simulink model "accel_test"  (R2022a)
settings: Solver=VariableStepAuto  StartTime=0.0  StopTime=10.0  RelTol=1e-3
values from neighbouring files (symbols this model uses):
  nx = 12 + 2*n    [nmpc_matlab.m]    (also in nmpc_test.m)
  ny = 8    [nmpc_matlab.m]    (also in nmpc_test.m)
  q_dot_0 = zeros(N, 1)    [ee_dyn_check.m]
  tau = [taub; taum]    [ee_dyn_check.m]
undefined symbols (not defined in the file or in its folder): fx, fy, fz, nz, q_0
settings Model: Creator=charl  LastModifiedBy=charl

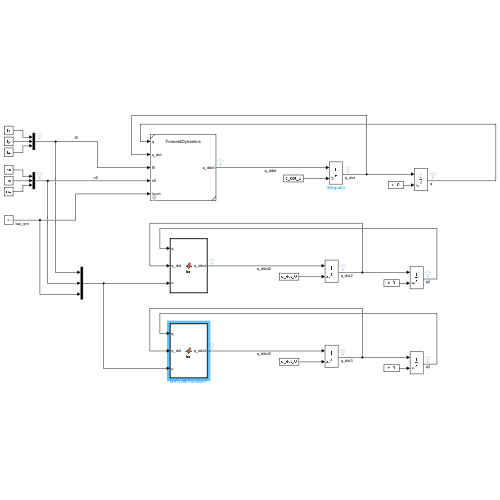
[thumbnail: Simulink's stored preview of the top-level diagram]
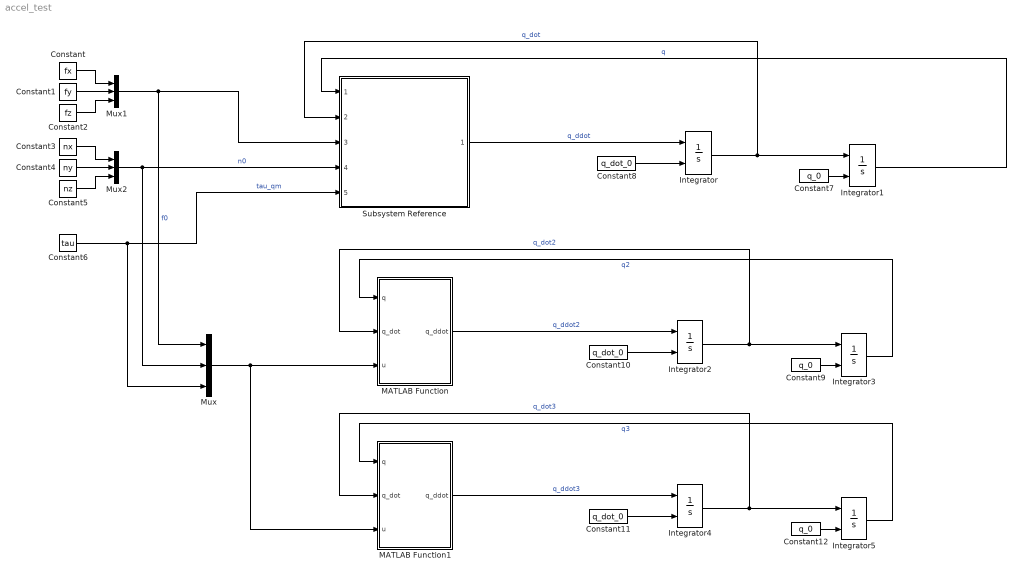
== system accel_test ==
  Constant : Constant  Value=fx
  Constant1 : Constant  Value=fy
  Constant10 : Constant  Value=q_dot_0
  Constant11 : Constant  Value=q_dot_0
  Constant12 : Constant  Value=q_0
  Constant2 : Constant  Value=fz
  Constant3 : Constant  Value=nx
  Constant4 : Constant  Value=ny
  Constant5 : Constant  Value=nz
  Constant6 : Constant  Value=tau
  Constant7 : Constant  Value=q_0
  Constant8 : Constant  Value=q_dot_0
  Constant9 : Constant  Value=q_0
  Integrator{,1..5} (6 alike) : Integrator  InitialConditionSource=external
  MATLAB Function : MATLAB Function  TreatAsAtomicUnit=on
  MATLAB Function1 : MATLAB Function  TreatAsAtomicUnit=on
  Mux : Mux  Inputs=3
  Mux1 : Mux  Inputs=3
  Mux2 : Mux  Inputs=3
  Subsystem Reference : Subsystem  ReferencedSubsystem=ForwardDynamics  spaceRobot=sr  SimulateUsing=Interpreted execution
  wires:
  Integrator/1 -> Subsystem Reference/2, Integrator1/1  "q_dot"
  Integrator1/1 -> Subsystem Reference/1  "q"
  Constant7/1 -> Integrator1/2
  Constant8/1 -> Integrator/2
  Subsystem Reference/1 -> Integrator/1  "q_ddot"
  Mux1/1 -> Mux/1, Subsystem Reference/3  "f0"
  Constant4/1 -> Mux2/2
  Mux2/1 -> Mux/2, Subsystem Reference/4  "n0"
  Constant/1 -> Mux1/1
  Constant6/1 -> Mux/3, Subsystem Reference/5  "tau_qm"
  Constant2/1 -> Mux1/3
  Constant1/1 -> Mux1/2
  Constant3/1 -> Mux2/1
  Constant5/1 -> Mux2/3
  MATLAB Function/1(q_ddot) -> Integrator2/1  "q_ddot2"
  Constant9/1 -> Integrator3/2
  Integrator2/1 -> MATLAB Function/2(q_dot), Integrator3/1  "q_dot2"
  Integrator3/1 -> MATLAB Function/1(q)  "q2"
  Constant10/1 -> Integrator2/2
  Constant12/1 -> Integrator5/2
  MATLAB Function1/1(q_ddot) -> Integrator4/1  "q_ddot3"
  Integrator5/1 -> MATLAB Function1/1(q)  "q3"
  Mux/1 -> MATLAB Function1/3(u), MATLAB Function/3(u)
  Constant11/1 -> Integrator4/2
  Integrator4/1 -> MATLAB Function1/2(q_dot), Integrator5/1  "q_dot3"

== matlab function accel_test/MATLAB Function1 ==
  data: q input; q_ddot output; q_dot input; u input
function q_ddot = fcn(q, q_dot, u)

%% Load params
sr_info = SR2_info();

%%
% 1 - Kinematics
[Rb, Ra, Rm] = RFunc_SR2(q);
Rm = reshape(Rm, 3, 3, []); % Split Rm to nk 3x3 arrays

% 2 - Kinetics
[t, ~, Omega, A, A_dot] = Kin(sr_info, q, q_dot, zeros(8, 1), {Rb, Ra, Rm});

% 3 - ID  
wb = t{1}(4:6);
C = CorMat(sr_info, wb, Omega, A, A_dot, {Rb, Ra, Rm});
h = C*q_dot;

% 4 - Mass Mat
D = MassM(sr_info, q, A);

% 5 - FD
q_ddot = D^ - 1 * (u - h);

== matlab function accel_test/MATLAB Function ==
  data: q input; q_ddot output; q_dot input; u input
function q_ddot = fcn(q, q_dot, u)

%% Load params
sr_info = SR2_info();

%%
% 1 - Kinematics
[Rb, Ra, Rm] = RFunc_SR2(q);
Rm = reshape(Rm, 3, 3, []); % Split Rm to nk 3x3 arrays

% 2 - Kinetics
[t, t_dot, Omega, A, A_dot] = Kin(sr_info, q, q_dot, zeros(8, 1), {Rb, Ra, Rm});

% 3 - ID  
[tau, ~] = ID(sr_info, t, t_dot, Omega, A, A_dot);
tau_b = blkdiag(Rb, zeros(3, 3)) * tau{1}; % Express base torque in intertial frame
h = [tau_b; tau{2}];

% 4 - Mass Mat
D = MassM(sr_info, q, A);

% 5 - FD
q_ddot = D^ - 1 * (u - h);
